simulink model "inversor_no_ideal_desag"  (R2023b)
settings: Solver=VariableStepAuto  StartTime=0.0  StopTime=10.0  RelTol=1e-3
undefined symbols (not defined in the file or in its folder): K_v_amort, K_v_wn2, V_sat_max, V_sat_min, X0_va, X0_vb, X0_vc
settings Model: Creator=Pc  LastModifiedBy=Gabriel

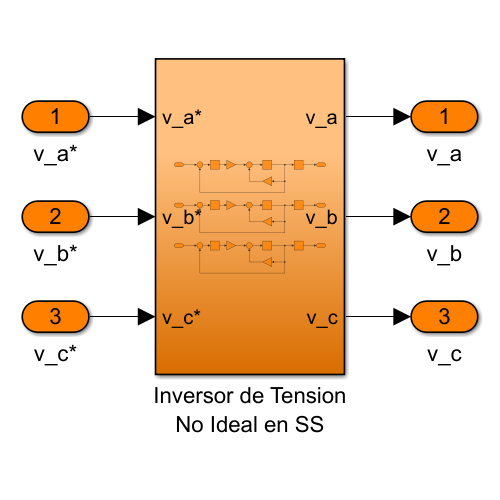
[thumbnail: Simulink's stored preview of the top-level diagram]
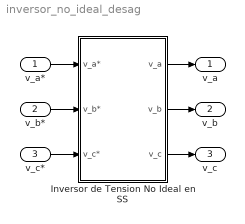
== system inversor_no_ideal_desag ==
  v_a* : Inport
  v_b* : Inport  Port=2
  v_c* : Inport  Port=3
  Inversor de Tension No Ideal en SS : Subsystem
  v_a : Outport
  v_b : Outport  Port=2
  v_c : Outport  Port=3
  wires:
  v_a*/1 -> Inversor de Tension No Ideal en SS/1(v_a*)
  v_b*/1 -> Inversor de Tension No Ideal en SS/2(v_b*)
  v_c*/1 -> Inversor de Tension No Ideal en SS/3(v_c*)
  Inversor de Tension No Ideal en SS/1(v_a) -> v_a/1
  Inversor de Tension No Ideal en SS/2(v_b) -> v_b/1
  Inversor de Tension No Ideal en SS/3(v_c) -> v_c/1

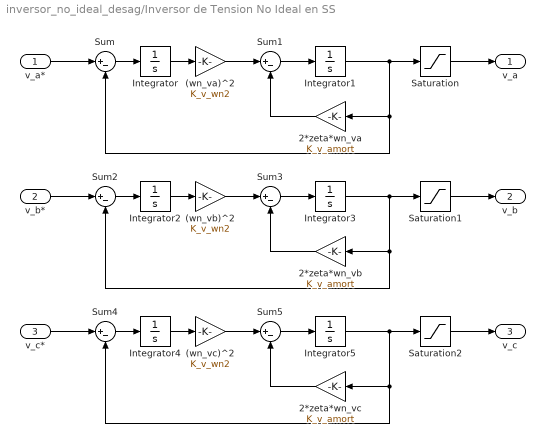
== system inversor_no_ideal_desag/Inversor de Tension No Ideal en SS ==
  v_a* : Inport
  v_b* : Inport  Port=2
  v_c* : Inport  Port=3
  (wn_va)^2 : Gain  Gain=K_v_wn2
  (wn_vb)^2 : Gain  Gain=K_v_wn2
  (wn_vc)^2 : Gain  Gain=K_v_wn2
  2*zeta*wn_va : Gain  Gain=K_v_amort
  2*zeta*wn_vb : Gain  Gain=K_v_amort
  2*zeta*wn_vc : Gain  Gain=K_v_amort
  Integrator : Integrator  InitialCondition=X0_va(1)
  Integrator1 : Integrator  InitialCondition=X0_va(2)
  Integrator2 : Integrator  InitialCondition=X0_vb(1)
  Integrator3 : Integrator  InitialCondition=X0_vb(2)
  Integrator4 : Integrator  InitialCondition=X0_vc(1)
  Integrator5 : Integrator  InitialCondition=X0_vc(2)
  Saturation : Saturate  UpperLimit=V_sat_max  LowerLimit=V_sat_min
  Saturation1 : Saturate  UpperLimit=V_sat_max  LowerLimit=V_sat_min
  Saturation2 : Saturate  UpperLimit=V_sat_max  LowerLimit=V_sat_min
  Sum{,1..5} (6 alike) : Sum  Inputs=|+-
  v_a : Outport
  v_b : Outport  Port=2
  v_c : Outport  Port=3
  wires:
  Saturation1/1 -> v_b/1
  Saturation/1 -> v_a/1
  Saturation2/1 -> v_c/1
  Sum/1 -> Integrator/1
  v_a*/1 -> Sum/1
  (wn_va)^2/1 -> Sum1/1
  2*zeta*wn_va/1 -> Sum1/2
  Sum1/1 -> Integrator1/1
  Integrator1/1 -> 2*zeta*wn_va/1, Sum/2, Saturation/1
  Integrator/1 -> (wn_va)^2/1
  Integrator2/1 -> (wn_vb)^2/1
  Integrator3/1 -> Saturation1/1, Sum2/2, 2*zeta*wn_vb/1
  Sum3/1 -> Integrator3/1
  2*zeta*wn_vb/1 -> Sum3/2
  (wn_vb)^2/1 -> Sum3/1
  Sum2/1 -> Integrator2/1
  v_b*/1 -> Sum2/1
  Sum4/1 -> Integrator4/1
  (wn_vc)^2/1 -> Sum5/1
  2*zeta*wn_vc/1 -> Sum5/2
  Sum5/1 -> Integrator5/1
  Integrator5/1 -> Saturation2/1, 2*zeta*wn_vc/1, Sum4/2
  Integrator4/1 -> (wn_vc)^2/1
  v_c*/1 -> Sum4/1
